simulink model "MPC_stateflow"  (R2018b)
settings: Solver=ode4  StartTime=0.0  StopTime=10  FixedStep=0.01  RelTol=1e-3
values from neighbouring files (symbols this model uses):
  bx0 = 0.4*rand - 0.2    [DataCollection_TrainMPC.m]
  by0 = 0.4*rand - 0.2    [DataCollection_TrainMPC.m]
  bz0 = 0.4*rand - 0.2    [DataCollection_TrainMPC.m]
  px0 = bx0 - (0.1*rand - 0.05)    [DataCollection_TrainMPC.m]
  py0 = by0 - (0.1*rand - 0.05)    [DataCollection_TrainMPC.m]
libraries: neural x148
(part 2 of 5)

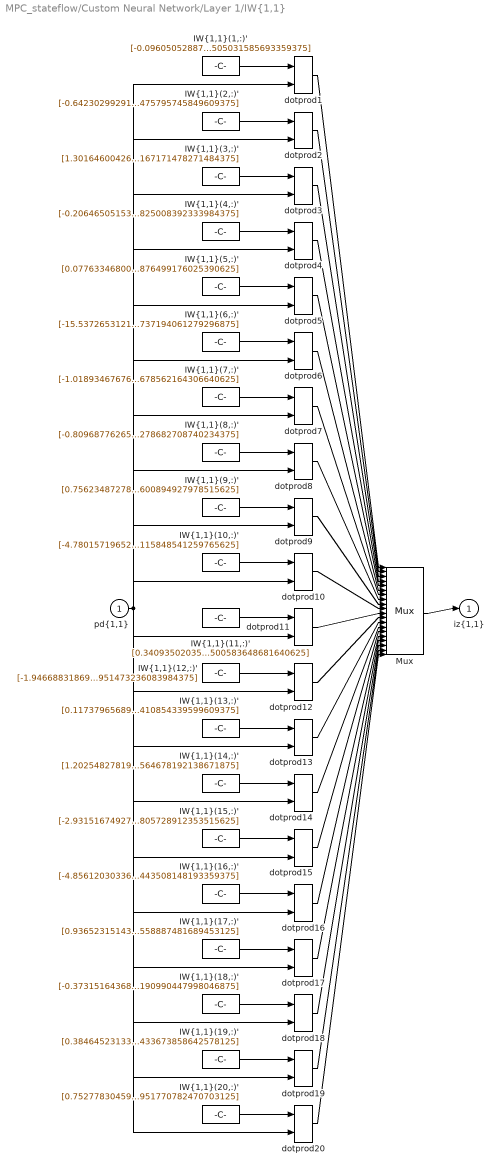
== system MPC_stateflow/Custom Neural Network/Layer 1/IW{1,1} ==
  "pd{1,1}" : Inport  PortDimensions=6
      mask Display: e = 0.06;c1 = [120 230 180]/255;c2 = ([120 230 180]+0)/(256+128);c3 = ([120 230 180]+128)/(256+128);patch([0 1 1 0],[0 0 1 1],c1);patch([0 1 1 1-e 1-e 0+e],[0 0 1 1-e 0+e 0+e],c2);patch([0 0 1 1-e 0+e 0+e],[0 1 1 1-e 1-e 0+e],c3);plot([0 1 1 0 0],[0 0 1 1 0]);
  "IW{1,1}(1,:)'" : Constant  Value=[-0.0960505288717609373438932607314200140535831451416015625;0.831752486119598177793932336498983204364776611328125;-0.0022915027448587575210903199973699884139932692050933837890625;1.253737241349362374620568516547791659832000732421875;1.745603804794473301598145553725771605968475341796875;0.98904804187790629210752513245097361505031585693359375]
      mask Display: e = 0.06;c1 = [120 150 230]/255;c2 = ([120 150 230]+0)/383;c3 = ([120 150 230]+128)/383;patch([0 1 1 0],[0 0 1 1],c1);patch([0 1 1 1-e 1-e 0+e],[0 0 1 1-e 0+e 0+e],c2);patch([0 0 1 1-e 0+e 0+e],[0 1 1 1-e 1-e 0+e],c3);plot([0 1 1 0 0],[0 0 1 1 0]);disp('Weights');
  "IW{1,1}(10,:)'" : Constant  Value=[-4.78015719652584802901174043654464185237884521484375;1.82750965351689753646269309683702886104583740234375;-0.44913035065545636737027734852745197713375091552734375;-0.296705961738857049159179268826846964657306671142578125;1.0273367507350636973484370173537172377109527587890625;-0.76732559429883784307691030335263349115848541259765625]
      mask Display: e = 0.06;c1 = [120 150 230]/255;c2 = ([120 150 230]+0)/383;c3 = ([120 150 230]+128)/383;patch([0 1 1 0],[0 0 1 1],c1);patch([0 1 1 1-e 1-e 0+e],[0 0 1 1-e 0+e 0+e],c2);patch([0 0 1 1-e 0+e 0+e],[0 1 1 1-e 1-e 0+e],c3);plot([0 1 1 0 0],[0 0 1 1 0]);disp('Weights');
  "IW{1,1}(11,:)'" : Constant  Value=[0.3409350203568044523905200549052096903324127197265625;-0.368968737987874106920571648515760898590087890625;-0.8932749097658392312126807155436836183071136474609375;-0.66929160576613444533222718746401369571685791015625;-0.5259460395139445854084669917938299477100372314453125;0.510926105204932756720381803461350500583648681640625]
      mask Display: e = 0.06;c1 = [120 150 230]/255;c2 = ([120 150 230]+0)/383;c3 = ([120 150 230]+128)/383;patch([0 1 1 0],[0 0 1 1],c1);patch([0 1 1 1-e 1-e 0+e],[0 0 1 1-e 0+e 0+e],c2);patch([0 0 1 1-e 0+e 0+e],[0 1 1 1-e 1-e 0+e],c3);plot([0 1 1 0 0],[0 0 1 1 0]);disp('Weights');
  "IW{1,1}(12,:)'" : Constant  Value=[-1.94668831869893121933046131744049489498138427734375;1.8928403055050029291095370354014448821544647216796875;-0.79762269677632680053847025192226283252239227294921875;1.724573381713232489431675276136957108974456787109375;1.37021376275906714425900645437650382518768310546875;-1.2105960555774204490120382615714333951473236083984375]
      mask Display: e = 0.06;c1 = [120 150 230]/255;c2 = ([120 150 230]+0)/383;c3 = ([120 150 230]+128)/383;patch([0 1 1 0],[0 0 1 1],c1);patch([0 1 1 1-e 1-e 0+e],[0 0 1 1-e 0+e 0+e],c2);patch([0 0 1 1-e 0+e 0+e],[0 1 1 1-e 1-e 0+e],c3);plot([0 1 1 0 0],[0 0 1 1 0]);disp('Weights');
  "IW{1,1}(13,:)'" : Constant  Value=[0.1173796568915033144975268442067317664623260498046875;0.6692513437947458232457620397326536476612091064453125;-0.7065428501883797007820930957677774131298065185546875;-0.3044682805089868882220116574899293482303619384765625;0.1473589733445717087079174234531819820404052734375;0.8460490710929666757778022656566463410854339599609375]
      mask Display: e = 0.06;c1 = [120 150 230]/255;c2 = ([120 150 230]+0)/383;c3 = ([120 150 230]+128)/383;patch([0 1 1 0],[0 0 1 1],c1);patch([0 1 1 1-e 1-e 0+e],[0 0 1 1-e 0+e 0+e],c2);patch([0 0 1 1-e 0+e 0+e],[0 1 1 1-e 1-e 0+e],c3);plot([0 1 1 0 0],[0 0 1 1 0]);disp('Weights');
  "IW{1,1}(14,:)'" : Constant  Value=[1.20254827819926735088529312633909285068511962890625;-2.1065505856942312590263099991716444492340087890625;0.66666924060894905412766320296213962137699127197265625;0.0902543188752378544581489450138178654015064239501953125;-1.3922068727151548639398015438928268849849700927734375;0.9483720525673191570348308232496492564678192138671875]
      mask Display: e = 0.06;c1 = [120 150 230]/255;c2 = ([120 150 230]+0)/383;c3 = ([120 150 230]+128)/383;patch([0 1 1 0],[0 0 1 1],c1);patch([0 1 1 1-e 1-e 0+e],[0 0 1 1-e 0+e 0+e],c2);patch([0 0 1 1-e 0+e 0+e],[0 1 1 1-e 1-e 0+e],c3);plot([0 1 1 0 0],[0 0 1 1 0]);disp('Weights');
  "IW{1,1}(15,:)'" : Constant  Value=[-2.931516749274532873670295884949155151844024658203125;0.94843863218748136745261945179663598537445068359375;1.0367786200063264789861250392277725040912628173828125;0.6904689270590800287408228541607968509197235107421875;1.0261103722150346495567418969585560262203216552734375;0.81446211351128694477807812290848232805728912353515625]
      mask Display: e = 0.06;c1 = [120 150 230]/255;c2 = ([120 150 230]+0)/383;c3 = ([120 150 230]+128)/383;patch([0 1 1 0],[0 0 1 1],c1);patch([0 1 1 1-e 1-e 0+e],[0 0 1 1-e 0+e 0+e],c2);patch([0 0 1 1-e 0+e 0+e],[0 1 1 1-e 1-e 0+e],c3);plot([0 1 1 0 0],[0 0 1 1 0]);disp('Weights');
  "IW{1,1}(16,:)'" : Constant  Value=[-4.856120303363926637985059642232954502105712890625;2.2395310961634660174013333744369447231292724609375;-0.74952380593419498655549659815733321011066436767578125;-1.9575546016491471856824091446469537913799285888671875;-0.49184046909802692226776343886740505695343017578125;0.044504062701382872402344759166226140223443508148193359375]
      mask Display: e = 0.06;c1 = [120 150 230]/255;c2 = ([120 150 230]+0)/383;c3 = ([120 150 230]+128)/383;patch([0 1 1 0],[0 0 1 1],c1);patch([0 1 1 1-e 1-e 0+e],[0 0 1 1-e 0+e 0+e],c2);patch([0 0 1 1-e 0+e 0+e],[0 1 1 1-e 1-e 0+e],c3);plot([0 1 1 0 0],[0 0 1 1 0]);disp('Weights');
  "IW{1,1}(17,:)'" : Constant  Value=[0.936523151438795053991270833648741245269775390625;0.4963313087596787909205886535346508026123046875;-0.1718880243608633673346730574849061667919158935546875;0.247344414111217769658424003864638507366180419921875;0.05411620451521859109789147623814642429351806640625;-0.9475780262445614443578278951463289558887481689453125]
      mask Display: e = 0.06;c1 = [120 150 230]/255;c2 = ([120 150 230]+0)/383;c3 = ([120 150 230]+128)/383;patch([0 1 1 0],[0 0 1 1],c1);patch([0 1 1 1-e 1-e 0+e],[0 0 1 1-e 0+e 0+e],c2);patch([0 0 1 1-e 0+e 0+e],[0 1 1 1-e 1-e 0+e],c3);plot([0 1 1 0 0],[0 0 1 1 0]);disp('Weights');
  "IW{1,1}(18,:)'" : Constant  Value=[-0.37315164368151432228160047088749706745147705078125;-0.4391120158711896426240173241239972412586212158203125;0.3888003154554902085493495178525336086750030517578125;0.501884868054674360138278643717058002948760986328125;0.771884198621549000307595633785240352153778076171875;-0.94338702395841078640614796313457190990447998046875]
      mask Display: e = 0.06;c1 = [120 150 230]/255;c2 = ([120 150 230]+0)/383;c3 = ([120 150 230]+128)/383;patch([0 1 1 0],[0 0 1 1],c1);patch([0 1 1 1-e 1-e 0+e],[0 0 1 1-e 0+e 0+e],c2);patch([0 0 1 1-e 0+e 0+e],[0 1 1 1-e 1-e 0+e],c3);plot([0 1 1 0 0],[0 0 1 1 0]);disp('Weights');
  "IW{1,1}(19,:)'" : Constant  Value=[0.38464523133862815740258156438358128070831298828125;0.578558656902977030966894744778983294963836669921875;-0.171641460946194701620015621301718056201934814453125;-0.3022033160443149402141216341988183557987213134765625;-0.2854604799950004601072350851609371602535247802734375;-0.5075778647939082066642413337831385433673858642578125]
      mask Display: e = 0.06;c1 = [120 150 230]/255;c2 = ([120 150 230]+0)/383;c3 = ([120 150 230]+128)/383;patch([0 1 1 0],[0 0 1 1],c1);patch([0 1 1 1-e 1-e 0+e],[0 0 1 1-e 0+e 0+e],c2);patch([0 0 1 1-e 0+e 0+e],[0 1 1 1-e 1-e 0+e],c3);plot([0 1 1 0 0],[0 0 1 1 0]);disp('Weights');
  "IW{1,1}(2,:)'" : Constant  Value=[-0.642302992918277748657374104368500411510467529296875;-0.84943356794090962846865977553534321486949920654296875;0.85502506496665431345860497458488680422306060791015625;0.1584127887998298678251529736371594481170177459716796875;-0.42114165791157687213086546762497164309024810791015625;0.3236613198298134985719798351055942475795745849609375]
      mask Display: e = 0.06;c1 = [120 150 230]/255;c2 = ([120 150 230]+0)/383;c3 = ([120 150 230]+128)/383;patch([0 1 1 0],[0 0 1 1],c1);patch([0 1 1 1-e 1-e 0+e],[0 0 1 1-e 0+e 0+e],c2);patch([0 0 1 1-e 0+e 0+e],[0 1 1 1-e 1-e 0+e],c3);plot([0 1 1 0 0],[0 0 1 1 0]);disp('Weights');
  "IW{1,1}(20,:)'" : Constant  Value=[0.752778304592076619172758000786416232585906982421875;-0.793547986844715946830319808213971555233001708984375;-0.9000930821078256816036855525453574955463409423828125;-0.460144216469947853198618759051896631717681884765625;0.817070301839598389648244847194291651248931884765625;0.7200558973657760208908484855783171951770782470703125]
      mask Display: e = 0.06;c1 = [120 150 230]/255;c2 = ([120 150 230]+0)/383;c3 = ([120 150 230]+128)/383;patch([0 1 1 0],[0 0 1 1],c1);patch([0 1 1 1-e 1-e 0+e],[0 0 1 1-e 0+e 0+e],c2);patch([0 0 1 1-e 0+e 0+e],[0 1 1 1-e 1-e 0+e],c3);plot([0 1 1 0 0],[0 0 1 1 0]);disp('Weights');
  "IW{1,1}(3,:)'" : Constant  Value=[1.301646004268869116771156768663786351680755615234375;-1.57046632470833369410456725745461881160736083984375;-0.049104865692711878455423146760949748568236827850341796875;0.231719255396934553647980692403507418930530548095703125;0.80525102346289945121071696121362037956714630126953125;0.800968281191005271324456771253608167171478271484375]
      mask Display: e = 0.06;c1 = [120 150 230]/255;c2 = ([120 150 230]+0)/383;c3 = ([120 150 230]+128)/383;patch([0 1 1 0],[0 0 1 1],c1);patch([0 1 1 1-e 1-e 0+e],[0 0 1 1-e 0+e 0+e],c2);patch([0 0 1 1-e 0+e 0+e],[0 1 1 1-e 1-e 0+e],c3);plot([0 1 1 0 0],[0 0 1 1 0]);disp('Weights');
  "IW{1,1}(4,:)'" : Constant  Value=[-0.20646505153866012705066168564371764659881591796875;-0.6603391608708621962620100021013058722019195556640625;-0.4244493228273025220431691195699386298656463623046875;0.8891895119816266568335549891344271600246429443359375;0.3268829956368961564550090770353563129901885986328125;0.381793835033847894777636611252091825008392333984375]
      mask Display: e = 0.06;c1 = [120 150 230]/255;c2 = ([120 150 230]+0)/383;c3 = ([120 150 230]+128)/383;patch([0 1 1 0],[0 0 1 1],c1);patch([0 1 1 1-e 1-e 0+e],[0 0 1 1-e 0+e 0+e],c2);patch([0 0 1 1-e 0+e 0+e],[0 1 1 1-e 1-e 0+e],c3);plot([0 1 1 0 0],[0 0 1 1 0]);disp('Weights');
  "IW{1,1}(5,:)'" : Constant  Value=[0.07763346800671389047465709154494106769561767578125;0.7562850068588262697488744379370473325252532958984375;-0.739942855763444651273630370269529521465301513671875;0.1731100810039858384214994657668285071849822998046875;0.243391440418243565346756440703757107257843017578125;0.9946457009029610052408543197088874876499176025390625]
      mask Display: e = 0.06;c1 = [120 150 230]/255;c2 = ([120 150 230]+0)/383;c3 = ([120 150 230]+128)/383;patch([0 1 1 0],[0 0 1 1],c1);patch([0 1 1 1-e 1-e 0+e],[0 0 1 1-e 0+e 0+e],c2);patch([0 0 1 1-e 0+e 0+e],[0 1 1 1-e 1-e 0+e],c3);plot([0 1 1 0 0],[0 0 1 1 0]);disp('Weights');
  "IW{1,1}(6,:)'" : Constant  Value=[-15.5372653121939325870926040806807577610015869140625;3.589611078180853009911288609146140515804290771484375;1.37647289136015427146730871754698455333709716796875;1.5003997535436688348653433422441594302654266357421875;-0.325500014040861429531759085875819437205791473388671875;-3.467041960174273906858388727414421737194061279296875]
      mask Display: e = 0.06;c1 = [120 150 230]/255;c2 = ([120 150 230]+0)/383;c3 = ([120 150 230]+128)/383;patch([0 1 1 0],[0 0 1 1],c1);patch([0 1 1 1-e 1-e 0+e],[0 0 1 1-e 0+e 0+e],c2);patch([0 0 1 1-e 0+e 0+e],[0 1 1 1-e 1-e 0+e],c3);plot([0 1 1 0 0],[0 0 1 1 0]);disp('Weights');
  "IW{1,1}(7,:)'" : Constant  Value=[-1.0189346767621552114491123575135134160518646240234375;0.1768304140142595570761585577201913110911846160888671875;0.322206858111667215904816430338541977107524871826171875;-1.202209597665699458701737967203371226787567138671875;0.73157917366419311644420986340264789760112762451171875;-0.61255466054129359410040933653363026678562164306640625]
      mask Display: e = 0.06;c1 = [120 150 230]/255;c2 = ([120 150 230]+0)/383;c3 = ([120 150 230]+128)/383;patch([0 1 1 0],[0 0 1 1],c1);patch([0 1 1 1-e 1-e 0+e],[0 0 1 1-e 0+e 0+e],c2);patch([0 0 1 1-e 0+e 0+e],[0 1 1 1-e 1-e 0+e],c3);plot([0 1 1 0 0],[0 0 1 1 0]);disp('Weights');
  "IW{1,1}(8,:)'" : Constant  Value=[-0.80968776265257436097755316950497217476367950439453125;0.248817525879779954944837072616792283952236175537109375;0.078067363609808093638520176682504825294017791748046875;-1.8628564188519332045501641914597712457180023193359375;0.06005555953149104009280989657781901769340038299560546875;-0.043826552099953862418058037064838572405278682708740234375]
      mask Display: e = 0.06;c1 = [120 150 230]/255;c2 = ([120 150 230]+0)/383;c3 = ([120 150 230]+128)/383;patch([0 1 1 0],[0 0 1 1],c1);patch([0 1 1 1-e 1-e 0+e],[0 0 1 1-e 0+e 0+e],c2);patch([0 0 1 1-e 0+e 0+e],[0 1 1 1-e 1-e 0+e],c3);plot([0 1 1 0 0],[0 0 1 1 0]);disp('Weights');
  "IW{1,1}(9,:)'" : Constant  Value=[0.756234872781890832271756153204478323459625244140625;0.0663305699460341458006951143033802509307861328125;-0.46890668125554757494910518289543688297271728515625;0.6147825774190476266767291235737502574920654296875;0.1567792287742635348735120714991353452205657958984375;0.3936363229798003349202417666674591600894927978515625]
      mask Display: e = 0.06;c1 = [120 150 230]/255;c2 = ([120 150 230]+0)/383;c3 = ([120 150 230]+128)/383;patch([0 1 1 0],[0 0 1 1],c1);patch([0 1 1 1-e 1-e 0+e],[0 0 1 1-e 0+e 0+e],c2);patch([0 0 1 1-e 0+e 0+e],[0 1 1 1-e 1-e 0+e],c3);plot([0 1 1 0 0],[0 0 1 1 0]);disp('Weights');
  Mux : Mux  Inputs=20
      mask Display: e = 0.06;c1 = [120 150 230]/255;c2 = ([120 150 230]+0)/383;c3 = ([120 150 230]+128)/383;patch([0 1 1 0],[0 0 1 1],c1);patch([0 1 1 1-e 1-e 0+e],[0 0 1 1-e 0+e 0+e],c2);patch([0 0 1 1-e 0+e 0+e],[0 1 1 1-e 1-e 0+e],c3);plot([0 1 1 0 0],[0 0 1 1 0]);disp('Mux');
  dotprod{1..20} (20 alike) : neural/Weight Functions/dotprod
  "iz{1,1}" : Outport
      mask Display: e = 0.06;c1 = [120 230 180]/255;c2 = ([120 230 180]+0)/(256+128);c3 = ([120 230 180]+128)/(256+128);patch([0 1 1 0],[0 0 1 1],c1);patch([0 1 1 1-e 1-e 0+e],[0 0 1 1-e 0+e 0+e],c2);patch([0 0 1 1-e 0+e 0+e],[0 1 1 1-e 1-e 0+e],c3);plot([0 1 1 0 0],[0 0 1 1 0]);
  wires:
  Mux/1 -> "iz{1,1}"/1
  dotprod20/1 -> Mux/20
  "IW{1,1}(20,:)'"/1 -> dotprod20/1
  dotprod19/1 -> Mux/19
  "IW{1,1}(19,:)'"/1 -> dotprod19/1
  dotprod18/1 -> Mux/18
  "IW{1,1}(18,:)'"/1 -> dotprod18/1
  dotprod17/1 -> Mux/17
  "IW{1,1}(17,:)'"/1 -> dotprod17/1
  dotprod16/1 -> Mux/16
  "IW{1,1}(16,:)'"/1 -> dotprod16/1
  dotprod15/1 -> Mux/15
  "IW{1,1}(15,:)'"/1 -> dotprod15/1
  dotprod14/1 -> Mux/14
  "IW{1,1}(14,:)'"/1 -> dotprod14/1
  dotprod13/1 -> Mux/13
  "IW{1,1}(13,:)'"/1 -> dotprod13/1
  dotprod12/1 -> Mux/12
  "IW{1,1}(12,:)'"/1 -> dotprod12/1
  dotprod11/1 -> Mux/11
  "IW{1,1}(11,:)'"/1 -> dotprod11/1
  dotprod10/1 -> Mux/10
  "IW{1,1}(10,:)'"/1 -> dotprod10/1
  dotprod9/1 -> Mux/9
  "IW{1,1}(9,:)'"/1 -> dotprod9/1
  dotprod8/1 -> Mux/8
  "IW{1,1}(8,:)'"/1 -> dotprod8/1
  dotprod7/1 -> Mux/7
  "IW{1,1}(7,:)'"/1 -> dotprod7/1
  dotprod6/1 -> Mux/6
  "IW{1,1}(6,:)'"/1 -> dotprod6/1
  dotprod5/1 -> Mux/5
  "IW{1,1}(5,:)'"/1 -> dotprod5/1
  dotprod4/1 -> Mux/4
  "IW{1,1}(4,:)'"/1 -> dotprod4/1
  dotprod3/1 -> Mux/3
  "IW{1,1}(3,:)'"/1 -> dotprod3/1
  dotprod2/1 -> Mux/2
  "IW{1,1}(2,:)'"/1 -> dotprod2/1
  dotprod1/1 -> Mux/1
  "pd{1,1}"/1 -> dotprod20/2, dotprod19/2, dotprod18/2, dotprod17/2, dotprod16/2, dotprod15/2, dotprod14/2, dotprod13/2, dotprod12/2, dotprod11/2, dotprod10/2, dotprod9/2, dotprod8/2, dotprod7/2, dotprod6/2, dotprod5/2, dotprod4/2, dotprod3/2, dotprod2/2, dotprod1/2
  "IW{1,1}(1,:)'"/1 -> dotprod1/1

== system MPC_stateflow/Custom Neural Network/Layer 2/Delays 1 ==
  "p{2}" : Inport  PortDimensions=20
      mask Display: e = 0.06;c1 = [120 230 180]/255;c2 = ([120 230 180]+0)/(256+128);c3 = ([120 230 180]+128)/(256+128);patch([0 1 1 0],[0 0 1 1],c1);patch([0 1 1 1-e 1-e 0+e],[0 0 1 1-e 0+e 0+e],c2);patch([0 0 1 1-e 0+e 0+e],[0 1 1 1-e 1-e 0+e],c3);plot([0 1 1 0 0],[0 0 1 1 0]);
  mux : Mux  Inputs=1
      mask Display: e = 0.06;c1 = [120 150 230]/255;c2 = ([120 150 230]+0)/383;c3 = ([120 150 230]+128)/383;patch([0 1 1 0],[0 0 1 1],c1);patch([0 1 1 1-e 1-e 0+e],[0 0 1 1-e 0+e 0+e],c2);patch([0 0 1 1-e 0+e 0+e],[0 1 1 1-e 1-e 0+e],c3);plot([0 1 1 0 0],[0 0 1 1 0]);disp('Mux')
  "pd{2,1}" : Outport
      mask Display: e = 0.06;c1 = [120 230 180]/255;c2 = ([120 230 180]+0)/(256+128);c3 = ([120 230 180]+128)/(256+128);patch([0 1 1 0],[0 0 1 1],c1);patch([0 1 1 1-e 1-e 0+e],[0 0 1 1-e 0+e 0+e],c2);patch([0 0 1 1-e 0+e 0+e],[0 1 1 1-e 1-e 0+e],c3);plot([0 1 1 0 0],[0 0 1 1 0]);
  wires:
  mux/1 -> "pd{2,1}"/1
  "p{2}"/1 -> mux/1

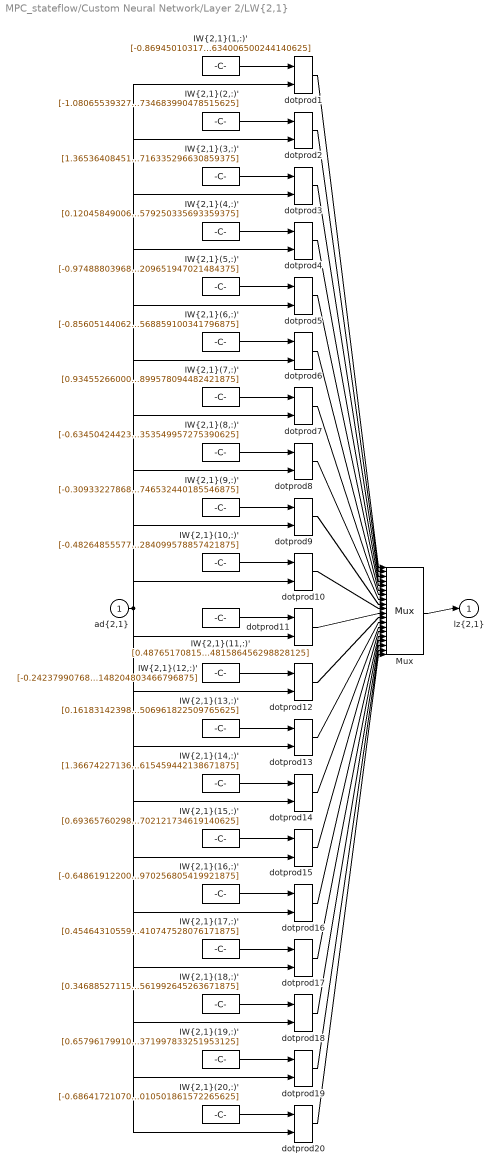
== system MPC_stateflow/Custom Neural Network/Layer 2/LW{2,1} ==
  "ad{2,1}" : Inport  PortDimensions=20
      mask Display: e = 0.06;c1 = [120 230 180]/255;c2 = ([120 230 180]+0)/(256+128);c3 = ([120 230 180]+128)/(256+128);patch([0 1 1 0],[0 0 1 1],c1);patch([0 1 1 1-e 1-e 0+e],[0 0 1 1-e 0+e 0+e],c2);patch([0 0 1 1-e 0+e 0+e],[0 1 1 1-e 1-e 0+e],c3);plot([0 1 1 0 0],[0 0 1 1 0]);
  "IW{2,1}(1,:)'" : Constant  Value=[-0.86945010317003645905487019263091497123241424560546875;-0.9628475956451809647518302881508134305477142333984375;0.464455301408056853151862242157221771776676177978515625;-0.0280186658061805093922203013789840042591094970703125;0.8802149646667343230177493751398287713527679443359375;2.19162758262292101107959751971065998077392578125;-0.2425698325555674383924298354031634517014026641845703125;1.201049187585670363631606960552744567394256591796875;-0.066239954473387374633830404491163790225982666015625;0.369904737379096015814639031304977834224700927734375;0.302608664681982109101454625488258898258209228515625;-0.25611748352890473245935254453797824680805206298828125;-0.4756538324541761397767913877032697200775146484375;1.1118975747010628740696347449556924402713775634765625;-0.66161830384654274350708647034480236470699310302734375;1.1658155789450137529428275229292921721935272216796875;-0.3788254964115800316193372054840438067913055419921875;0.256618075042714277600452987826429307460784912109375;-0.1728271699976773323470524701406247913837432861328125;-0.9351473493710857898264521281816996634006500244140625]
      mask Display: e = 0.06;c1 = [120 150 230]/255;c2 = ([120 150 230]+0)/383;c3 = ([120 150 230]+128)/383;patch([0 1 1 0],[0 0 1 1],c1);patch([0 1 1 1-e 1-e 0+e],[0 0 1 1-e 0+e 0+e],c2);patch([0 0 1 1-e 0+e 0+e],[0 1 1 1-e 1-e 0+e],c3);plot([0 1 1 0 0],[0 0 1 1 0]);disp('weights');
  "IW{2,1}(10,:)'" : Constant  Value=[-0.4826485557719604191362350320559926331043243408203125;-0.531652960170728494659897478413768112659454345703125;1.0598735632520319693838928287732414901256561279296875;-0.7298416839065373640238476582453586161136627197265625;-0.0194929547601445651849871865124441683292388916015625;-0.2250838339207545946152322358102537691593170166015625;0.2295412356918559992902117983248899690806865692138671875;0.2849397026270452659701959419180639088153839111328125;-0.6140745359617743037716763865319080650806427001953125;-0.054128823357529838589119464131726999767124652862548828125;0.2646066348602555962088445085100829601287841796875;-0.94862699481696888259563138490193523466587066650390625;0.1868648989292420736774147371761500835418701171875;0.715345962889761377567765521234832704067230224609375;-0.04799395507758442980250634946060017682611942291259765625;-0.27793384682627542137112186537706293165683746337890625;0.8777729547394266251814087809179909527301788330078125;-0.2574124774418911076878657695488072931766510009765625;0.32820511070958691135501794633455574512481689453125;0.648475679248995628967122684116475284099578857421875]
      mask Display: e = 0.06;c1 = [120 150 230]/255;c2 = ([120 150 230]+0)/383;c3 = ([120 150 230]+128)/383;patch([0 1 1 0],[0 0 1 1],c1);patch([0 1 1 1-e 1-e 0+e],[0 0 1 1-e 0+e 0+e],c2);patch([0 0 1 1-e 0+e 0+e],[0 1 1 1-e 1-e 0+e],c3);plot([0 1 1 0 0],[0 0 1 1 0]);disp('weights');
  "IW{2,1}(11,:)'" : Constant  Value=[0.4876517081501858807968119435827247798442840576171875;0.4906688618130041756870696190162561833858489990234375;0.8639441383936745655347522188094444572925567626953125;0.01132433135379340427562055992893874645233154296875;0.198220615291756718789883962017484009265899658203125;0.6576916159613859225174792300094850361347198486328125;0.3556017828686222070899702885071747004985809326171875;-0.863581303166591762732196002616547048091888427734375;-0.0008316586422278948731445780140347778797149658203125;-0.95533914401638764246627033571712672710418701171875;-0.309405076817836910407777395448647439479827880859375;-0.2669138055125113151433424718561582267284393310546875;0.6876808578623776480043261472019366919994354248046875;-0.315091760312960378342950207297690212726593017578125;-0.19521496028452833826349888113327324390411376953125;0.4636008182845905434277256063069216907024383544921875;-0.9381019874576985717595789537881501019001007080078125;0.8637222332730811746870358547312207520008087158203125;-0.005499813278937448757233141805045306682586669921875;0.2652316335559945503774770259042270481586456298828125]
      mask Display: e = 0.06;c1 = [120 150 230]/255;c2 = ([120 150 230]+0)/383;c3 = ([120 150 230]+128)/383;patch([0 1 1 0],[0 0 1 1],c1);patch([0 1 1 1-e 1-e 0+e],[0 0 1 1-e 0+e 0+e],c2);patch([0 0 1 1-e 0+e 0+e],[0 1 1 1-e 1-e 0+e],c3);plot([0 1 1 0 0],[0 0 1 1 0]);disp('weights');
  "IW{2,1}(12,:)'" : Constant  Value=[-0.2423799076801444185580436396776349283754825592041015625;0.71045454852867617745459938305430114269256591796875;-1.3972510679789784671100960622425191104412078857421875;-0.9569503894516040443107840474112890660762786865234375;-0.968933448898328553156034104176796972751617431640625;6.6339973785591297428254620172083377838134765625;-0.649974583994656018859359392081387341022491455078125;-0.420300460616720938933355000699521042406558990478515625;0.4571713359491924588695610509603284299373626708984375;0.345044005944761755788618984297499991953372955322265625;0.593177356014574996834198827855288982391357421875;1.492063845922114495579080539755523204803466796875;-0.2379677518755716203457950541633181273937225341796875;0.2460320798631776828546691149313119240105152130126953125;2.033348430009402907359117307350970804691314697265625;1.1844441437060206911979776123189367353916168212890625;0.4337573272633783449947486587916500866413116455078125;0.87373676261818733479458387591876089572906494140625;0.038031968147357542164854748989455401897430419921875;0.33746554041346410457435922580771148204803466796875]
      mask Display: e = 0.06;c1 = [120 150 230]/255;c2 = ([120 150 230]+0)/383;c3 = ([120 150 230]+128)/383;patch([0 1 1 0],[0 0 1 1],c1);patch([0 1 1 1-e 1-e 0+e],[0 0 1 1-e 0+e 0+e],c2);patch([0 0 1 1-e 0+e 0+e],[0 1 1 1-e 1-e 0+e],c3);plot([0 1 1 0 0],[0 0 1 1 0]);disp('weights');
  "IW{2,1}(13,:)'" : Constant  Value=[0.1618314239819113875551437331523629836738109588623046875;-0.470160884674381218673033799859695136547088623046875;-0.53793919689711755527383729713619686663150787353515625;0.8959404224353619827780903506209142506122589111328125;0.1869628163932743891706422800780273973941802978515625;0.253487772309714698426574841505498625338077545166015625;-0.1552545568891181282378255446019466035068035125732421875;-0.84467568268962833766266840029857121407985687255859375;-0.583611123182417035337721245014108717441558837890625;0.7376269640629706803025555927888490259647369384765625;-0.107707535993085468106755797634832561016082763671875;0.379956061558021251922667715916759334504604339599609375;0.499716621452286791082997297053225338459014892578125;-0.145456536333087027568211624384275637567043304443359375;-0.92896769722590288864694230142049491405487060546875;-0.202404310214908400578082137144519947469234466552734375;0.7820379085846778099977427700650878250598907470703125;0.688659897131426390615160926245152950286865234375;-0.6505596997821549987151001914753578603267669677734375;-0.046235332957613284321496394113637506961822509765625]
      mask Display: e = 0.06;c1 = [120 150 230]/255;c2 = ([120 150 230]+0)/383;c3 = ([120 150 230]+128)/383;patch([0 1 1 0],[0 0 1 1],c1);patch([0 1 1 1-e 1-e 0+e],[0 0 1 1-e 0+e 0+e],c2);patch([0 0 1 1-e 0+e 0+e],[0 1 1 1-e 1-e 0+e],c3);plot([0 1 1 0 0],[0 0 1 1 0]);disp('weights');
  "IW{2,1}(14,:)'" : Constant  Value=[1.366742271367725525266223485232330858707427978515625;-0.393363022776568704852451219267095439136028289794921875;0.35963396200540775904386237016296945512294769287109375;0.654230942341464949407736639841459691524505615234375;-0.1326473020210834352639039934729225933551788330078125;-3.28762404715274403343983067316003143787384033203125;-0.0911863455292211411151725997115136124193668365478515625;-0.350368599710001671354575591976754367351531982421875;-0.5039328832455385320798768589156679809093475341796875;0.509101395846049076254757892456836998462677001953125;0.5654988295683438526140207613934762775897979736328125;1.1192035066205392457305833886493928730487823486328125;0.022282956594256386750885212677530944347381591796875;0.10840420140515542868353549010862479917705059051513671875;0.96883348602309471431226484128274023532867431640625;-0.50278354234049416060514658965985290706157684326171875;-0.9454255529650623657289543189108371734619140625;0.8404130286113209447051985989673994481563568115234375;0.1414317030925127394169749095453880727291107177734375;-0.97372728615385550909877565572969615459442138671875]
      mask Display: e = 0.06;c1 = [120 150 230]/255;c2 = ([120 150 230]+0)/383;c3 = ([120 150 230]+128)/383;patch([0 1 1 0],[0 0 1 1],c1);patch([0 1 1 1-e 1-e 0+e],[0 0 1 1-e 0+e 0+e],c2);patch([0 0 1 1-e 0+e 0+e],[0 1 1 1-e 1-e 0+e],c3);plot([0 1 1 0 0],[0 0 1 1 0]);disp('weights');
  "IW{2,1}(15,:)'" : Constant  Value=[0.6936576029800705089911616596509702503681182861328125;-0.25983160417178741141697173588909208774566650390625;0.8980326413752328651440848261700011789798736572265625;-0.969962038515755242684690529131330549716949462890625;0.6147210577696828881499868657556362450122833251953125;0.1736666813121658936580615772982127964496612548828125;0.5952776079171331335970762665965594351291656494140625;-0.636774297338472461404990099254064261913299560546875;0.70334374987273395873899062280543148517608642578125;0.07688118518908737542005837894976139068603515625;0.9809435672476813916631499523646198213100433349609375;-0.6227263980893782413517101304023526608943939208984375;0.08190360992437728526738283107988536357879638671875;0.2529923172485875060289117755019105970859527587890625;-0.748717237724522366448809407302178442478179931640625;-0.653139658425754277004671166650950908660888671875;0.04410249450502146117969459737651050090789794921875;-0.544199420097366104442926371120847761631011962890625;0.993506850416419950988711207173764705657958984375;-0.2939878289163504465619780603446997702121734619140625]
      mask Display: e = 0.06;c1 = [120 150 230]/255;c2 = ([120 150 230]+0)/383;c3 = ([120 150 230]+128)/383;patch([0 1 1 0],[0 0 1 1],c1);patch([0 1 1 1-e 1-e 0+e],[0 0 1 1-e 0+e 0+e],c2);patch([0 0 1 1-e 0+e 0+e],[0 1 1 1-e 1-e 0+e],c3);plot([0 1 1 0 0],[0 0 1 1 0]);disp('weights');
  "IW{2,1}(16,:)'" : Constant  Value=[-0.64861912200991234112024130809004418551921844482421875;0.721480501821621711400212006992660462856292724609375;0.32699986582939588597440661033033393323421478271484375;-0.6476074888498895010258138427161611616611480712890625;-0.369510393809254100716543689486570656299591064453125;1.246805620640468514892518214765004813671112060546875;1.219610087621920246903073348221369087696075439453125;0.1662383984196948716327568718043039552867412567138671875;-0.1683025634649453206037605923484079539775848388671875;1.535647982148657941792180281481705605983734130859375;-0.3995033209321998679541820820304565131664276123046875;0.06036852059349755161843376072283717803657054901123046875;0.918868642123504830721003600046969950199127197265625;-1.2901867078027933199990684443037025630474090576171875;0.780400069817255737092409617616795003414154052734375;0.1990641497121203029596614442198188044130802154541015625;-0.34802037645994943204641458578407764434814453125;-0.8250355808928182543837692719534970819950103759765625;0.633670217583243822190297578345052897930145263671875;-0.0158563970128831055461660071159712970256805419921875]
      mask Display: e = 0.06;c1 = [120 150 230]/255;c2 = ([120 150 230]+0)/383;c3 = ([120 150 230]+128)/383;patch([0 1 1 0],[0 0 1 1],c1);patch([0 1 1 1-e 1-e 0+e],[0 0 1 1-e 0+e 0+e],c2);patch([0 0 1 1-e 0+e 0+e],[0 1 1 1-e 1-e 0+e],c3);plot([0 1 1 0 0],[0 0 1 1 0]);disp('weights');
  "IW{2,1}(17,:)'" : Constant  Value=[0.45464310559893561514144266766379587352275848388671875;0.4529374704014650365735406012390740215778350830078125;-0.75921684877630790655445025549852289259433746337890625;-0.33587285126632604459473441238515079021453857421875;0.785777417050302684486950965947471559047698974609375;9.3449961980014517592962874914519488811492919921875;1.6409870586549715198998455889523029327392578125;0.578457000499050355557528746430762112140655517578125;0.233370134310472376881762102129869163036346435546875;2.92359285650911271403629143605940043926239013671875;-0.7139883434838012465917245208402164280414581298828125;-0.10755020807965987028609333719941787421703338623046875;0.6079217829972936026905472317594103515148162841796875;-1.1541763575095778104895316573674790561199188232421875;1.0201769917919698560382357754861004650592803955078125;2.280579523437183286915796998073346912860870361328125;0.718978641731171652651255499222315847873687744140625;-0.54538052743062248595151686458848416805267333984375;0.1887452476619555508108305730274878442287445068359375;0.4601824221802086611887716571800410747528076171875]
      mask Display: e = 0.06;c1 = [120 150 230]/255;c2 = ([120 150 230]+0)/383;c3 = ([120 150 230]+128)/383;patch([0 1 1 0],[0 0 1 1],c1);patch([0 1 1 1-e 1-e 0+e],[0 0 1 1-e 0+e 0+e],c2);patch([0 0 1 1-e 0+e 0+e],[0 1 1 1-e 1-e 0+e],c3);plot([0 1 1 0 0],[0 0 1 1 0]);disp('weights');
  "IW{2,1}(18,:)'" : Constant  Value=[0.346885271156239516354702345779514871537685394287109375;0.348093907222798815137565497934701852500438690185546875;0.7381264553490314295203233996289782226085662841796875;-0.7380063103781662192659496213309466838836669921875;0.1557144305690709717993058802676387131214141845703125;2.367869383175240205474665344809181988239288330078125;-0.118973993123826726758807126316241919994354248046875;0.457037682108792753243875495172687806189060211181640625;-0.532667721521499881731642744853161275386810302734375;0.46675155999001127771208530248259194195270538330078125;0.80261687269854764537058144924230873584747314453125;1.451894766366281341873900601058267056941986083984375;-0.9353538667528520367255850942456163465976715087890625;-1.1424264474399457025555193467880599200725555419921875;0.1606066022159286232895425428068847395479679107666015625;-1.0421273903774366242913629321265034377574920654296875;0.11703310184503568081026969593949615955352783203125;-0.371246767771899133236956913606263697147369384765625;0.951978136661809859475624762126244604587554931640625;-0.0627433145077815890289230082998983561992645263671875]
      mask Display: e = 0.06;c1 = [120 150 230]/255;c2 = ([120 150 230]+0)/383;c3 = ([120 150 230]+128)/383;patch([0 1 1 0],[0 0 1 1],c1);patch([0 1 1 1-e 1-e 0+e],[0 0 1 1-e 0+e 0+e],c2);patch([0 0 1 1-e 0+e 0+e],[0 1 1 1-e 1-e 0+e],c3);plot([0 1 1 0 0],[0 0 1 1 0]);disp('weights');
  "IW{2,1}(19,:)'" : Constant  Value=[0.6579617991003574584141233572154305875301361083984375;-0.866927037291770119509237702004611492156982421875;0.2831324178926750700924230841337703168392181396484375;0.618981384253164179654049803502857685089111328125;-0.6319795967450698714884538276237435638904571533203125;0.3961144968946059830017247804789803922176361083984375;-0.4595834759404844316321714359219186007976531982421875;0.1389888254907514220093389667454175651073455810546875;-0.7960654811484051407433071290142834186553955078125;0.7082308876730774027663528613629750907421112060546875;0.0831187577747465322630660011782310903072357177734375;-0.5921875495337562966824407340027391910552978515625;0.418774502462590181295354341273196041584014892578125;-0.866550004721287070452717671287246048450469970703125;-0.9939640867608072749561642922344617545604705810546875;-0.47140503454619864243113624979741871356964111328125;0.380455736325495674776675514294765889644622802734375;-0.650468247287376843956963057280518114566802978515625;0.8031251693386425305476450375863350927829742431640625;-0.0851901678211366419901651170221157371997833251953125]
      mask Display: e = 0.06;c1 = [120 150 230]/255;c2 = ([120 150 230]+0)/383;c3 = ([120 150 230]+128)/383;patch([0 1 1 0],[0 0 1 1],c1);patch([0 1 1 1-e 1-e 0+e],[0 0 1 1-e 0+e 0+e],c2);patch([0 0 1 1-e 0+e 0+e],[0 1 1 1-e 1-e 0+e],c3);plot([0 1 1 0 0],[0 0 1 1 0]);disp('weights');
  "IW{2,1}(2,:)'" : Constant  Value=[-1.0806553932786810978683433859259821474552154541015625;-0.859955712561555341011398923001252114772796630859375;-0.81143099224970594018913061518105678260326385498046875;0.2086209658399464927924782386980950832366943359375;0.1640283598941600917697769546066410839557647705078125;-1.23271399361495515023534608189947903156280517578125;0.56672855173635083847472060369909740984439849853515625;0.48456887902243217514097750608925707638263702392578125;-0.309655897689570025477223680354654788970947265625;-0.6057893011983217501637000168557278811931610107421875;0.4070339763053059112252185514080338180065155029296875;0.12454988425188946721267058137527783401310443878173828125;0.50034482659598555898128324770368635654449462890625;-0.1687741106642130783921373904377105645835399627685546875;-1.359239838595867500004032990545965731143951416015625;0.82329734513879271329273024093708954751491546630859375;0.9648348985858856696751217896235175430774688720703125;-0.419806296625148345214029177441261708736419677734375;0.6327030236544282093547053591464646160602569580078125;-0.8128458083650385024299112046719528734683990478515625]
      mask Display: e = 0.06;c1 = [120 150 230]/255;c2 = ([120 150 230]+0)/383;c3 = ([120 150 230]+128)/383;patch([0 1 1 0],[0 0 1 1],c1);patch([0 1 1 1-e 1-e 0+e],[0 0 1 1-e 0+e 0+e],c2);patch([0 0 1 1-e 0+e 0+e],[0 1 1 1-e 1-e 0+e],c3);plot([0 1 1 0 0],[0 0 1 1 0]);disp('weights');
  "IW{2,1}(20,:)'" : Constant  Value=[-0.6864172107078314599704071952146477997303009033203125;-0.479369802842918080187928353552706539630889892578125;-0.2199845717175075154870000915252603590488433837890625;-0.3105266946334130917506399782723747193813323974609375;0.5758584676510085653688975071418099105358123779296875;0.7289588601091996356018398728338070213794708251953125;-0.4952665969908205401139866808080114424228668212890625;-0.678057126368782459024941999814473092555999755859375;0.0317140339370596269219504392822273075580596923828125;-0.802513196359303293547782232053577899932861328125;0.9494807417101644997359244371182285249233245849609375;-0.504534196475290297456695043365471065044403076171875;-0.0699970368729878611446793001960031688213348388671875;-0.0828323725831363599780843287589959800243377685546875;0.9023875709804090039511947907158173620700836181640625;0.638178357267061624469306480023078620433807373046875;-0.094293000096925094766220354358665645122528076171875;0.2141883239449209330729217981570400297641754150390625;0.1912158672052910457495045193354599177837371826171875;-0.7246745181087936860109266490326263010501861572265625]
      mask Display: e = 0.06;c1 = [120 150 230]/255;c2 = ([120 150 230]+0)/383;c3 = ([120 150 230]+128)/383;patch([0 1 1 0],[0 0 1 1],c1);patch([0 1 1 1-e 1-e 0+e],[0 0 1 1-e 0+e 0+e],c2);patch([0 0 1 1-e 0+e 0+e],[0 1 1 1-e 1-e 0+e],c3);plot([0 1 1 0 0],[0 0 1 1 0]);disp('weights');
  "IW{2,1}(3,:)'" : Constant  Value=[1.3653640845112018364915229540201835334300994873046875;0.306765011951229793485396157848299480974674224853515625;0.020793587999859898529653179366505355574190616607666015625;0.099095843017125151419577377964742481708526611328125;0.7576639688236881386984578057308681309223175048828125;3.3203980492572231497661050525493919849395751953125;0.051763083102982075656139926422838470898568630218505859375;0.341073559737574416583782976886141113936901092529296875;-0.5499200843718308195917643388384021818637847900390625;1.5318590406784975410658944383612833917140960693359375;0.22048162529325932013080091564916074275970458984375;0.820735541014840919160633347928524017333984375;-0.0860493451286143962164487675181590020656585693359375;-1.0167176992358555320805635346914641559123992919921875;1.6964552720312353617515555015415884554386138916015625;1.79534049531465367266491739428602159023284912109375;-0.466722595696729580794226421858184039592742919921875;-0.9813028440669684382413606726913712918758392333984375;-0.62973920346193867914053043932653963565826416015625;-0.869256569915547228077912222943268716335296630859375]
      mask Display: e = 0.06;c1 = [120 150 230]/255;c2 = ([120 150 230]+0)/383;c3 = ([120 150 230]+128)/383;patch([0 1 1 0],[0 0 1 1],c1);patch([0 1 1 1-e 1-e 0+e],[0 0 1 1-e 0+e 0+e],c2);patch([0 0 1 1-e 0+e 0+e],[0 1 1 1-e 1-e 0+e],c3);plot([0 1 1 0 0],[0 0 1 1 0]);disp('weights');
  "IW{2,1}(4,:)'" : Constant  Value=[0.1204584900671190894616557898189057596027851104736328125;-0.2802269618452044586121019165148027241230010986328125;0.2472333569965907695831219825777225196361541748046875;0.852362853412907295336253810091875493526458740234375;0.689468890784443733110720131662674248218536376953125;0.007761819150829019943460540531532387831248342990875244140625;-0.7987799736009602025177400719258002936840057373046875;0.5636780929170390752602770589874126017093658447265625;0.1850237375315935128838873424683697521686553955078125;-0.432454595119342533049433541236794553697109222412109375;0.5992305234720560758177043680916540324687957763671875;0.0219114806932921568627392616690485738217830657958984375;-0.886141123177810019484468284645117819309234619140625;-0.72251917139723842442577961264760233461856842041015625;-0.71985290991653083647605626538279466331005096435546875;-1.275377001876238924893414150574244558811187744140625;0.0673066899424228370918399377842433750629425048828125;0.153511869974181536235846579074859619140625;0.4037530595126208599054962178342975676059722900390625;-0.096533702617049410577010348788462579250335693359375]
      mask Display: e = 0.06;c1 = [120 150 230]/255;c2 = ([120 150 230]+0)/383;c3 = ([120 150 230]+128)/383;patch([0 1 1 0],[0 0 1 1],c1);patch([0 1 1 1-e 1-e 0+e],[0 0 1 1-e 0+e 0+e],c2);patch([0 0 1 1-e 0+e 0+e],[0 1 1 1-e 1-e 0+e],c3);plot([0 1 1 0 0],[0 0 1 1 0]);disp('weights');
  "IW{2,1}(5,:)'" : Constant  Value=[-0.9748880396817682925103554225643165409564971923828125;0.1377028741729626748480086462222971022129058837890625;0.8496159407987013967300526928738690912723541259765625;0.8374668712672121984041950781829655170440673828125;0.81078463741729844826977569027803838253021240234375;0.8372035559550516925497731790528632700443267822265625;-0.1783773001556288040347908463445492088794708251953125;0.4662850505750222307455032932921312749385833740234375;-0.3754603245961660729079767406801693141460418701171875;0.308274693941488653337046343949623405933380126953125;-0.9308575602567314977164869560510851442813873291015625;-0.729144193855660205372259952127933502197265625;0.0170324812204791786740543102496303617954254150390625;-0.1427623426724269339871398187824524939060211181640625;0.493876991215050242800543855992145836353302001953125;-0.684539860258933430259276065044105052947998046875;-0.37106597762830073605755387688986957073211669921875;-0.3771115717350743690161607446498237550258636474609375;-0.5192887503017222794454710310674272477626800537109375;-0.2491303336642844978854327564476989209651947021484375]
      mask Display: e = 0.06;c1 = [120 150 230]/255;c2 = ([120 150 230]+0)/383;c3 = ([120 150 230]+128)/383;patch([0 1 1 0],[0 0 1 1],c1);patch([0 1 1 1-e 1-e 0+e],[0 0 1 1-e 0+e 0+e],c2);patch([0 0 1 1-e 0+e 0+e],[0 1 1 1-e 1-e 0+e],c3);plot([0 1 1 0 0],[0 0 1 1 0]);disp('weights');
  "IW{2,1}(6,:)'" : Constant  Value=[-0.8560514406210264493068962110555730760097503662109375;-0.36527518135567849100198145606555044651031494140625;-0.473406459025778048044230672530829906463623046875;-0.21024877415289022764000037568621337413787841796875;-0.0802394683663860686095858909538947045803070068359375;-0.999195950217285133732048052479512989521026611328125;-0.197040833060918796348914838745258748531341552734375;0.0380232549281116494199750377447344362735748291015625;0.8326111069367014838604745818884111940860748291015625;-0.710908919750680379223695126711390912532806396484375;0.54047746910995986269199420348741114139556884765625;-0.2885896580322377946714595964294858276844024658203125;-0.576079670712648095332042430527508258819580078125;-0.7819624719618634145490432274527847766876220703125;-0.095190346507096901262912069796584546566009521484375;-0.6247366541951320240144696072093211114406585693359375;0.82154566234767489874002421856857836246490478515625;0.0345351970022595988751845652586780488491058349609375;0.1484381776817194076301120730931870639324188232421875;0.950700068540573095532408842700533568859100341796875]
      mask Display: e = 0.06;c1 = [120 150 230]/255;c2 = ([120 150 230]+0)/383;c3 = ([120 150 230]+128)/383;patch([0 1 1 0],[0 0 1 1],c1);patch([0 1 1 1-e 1-e 0+e],[0 0 1 1-e 0+e 0+e],c2);patch([0 0 1 1-e 0+e 0+e],[0 1 1 1-e 1-e 0+e],c3);plot([0 1 1 0 0],[0 0 1 1 0]);disp('weights');
  "IW{2,1}(7,:)'" : Constant  Value=[0.93455266000054404429420173983089625835418701171875;0.9772323088248977551728557955357246100902557373046875;-0.868077818631952435879384211148135364055633544921875;0.9265250568814236142856088918051682412624359130859375;0.09269363204074654305486546945758163928985595703125;0.953518298062119296076843966147862374782562255859375;-0.3652321080834461941577728794072754681110382080078125;0.5417678210037759622963449146482162177562713623046875;0.81927104990311416798931531957350671291351318359375;0.5030556342704877170746158299152739346027374267578125;0.4634572014790538929673857637681066989898681640625;-0.947562865407253429594902627286501228809356689453125;0.597208489520420382490328847779892385005950927734375;0.267573521223835708582328152260743081569671630859375;-0.0998265059984777547441581191378645598888397216796875;0.2449918045998422666542637671227566897869110107421875;-0.266886712297531136783845795434899628162384033203125;0.8328117061077955352033086455776356160640716552734375;-0.3020248055584222601765986837563104927539825439453125;-0.6640334136007701726356344806845299899578094482421875]
      mask Display: e = 0.06;c1 = [120 150 230]/255;c2 = ([120 150 230]+0)/383;c3 = ([120 150 230]+128)/383;patch([0 1 1 0],[0 0 1 1],c1);patch([0 1 1 1-e 1-e 0+e],[0 0 1 1-e 0+e 0+e],c2);patch([0 0 1 1-e 0+e 0+e],[0 1 1 1-e 1-e 0+e],c3);plot([0 1 1 0 0],[0 0 1 1 0]);disp('weights');
  "IW{2,1}(8,:)'" : Constant  Value=[-0.6345042442310167007946120065753348171710968017578125;-0.4717527842355411227259764928021468222141265869140625;0.788463567668844955704798849183134734630584716796875;-0.6520886666390712793628381405142135918140411376953125;0.5972071823040787652558947229408659040927886962890625;-3.374925678704658427164986278512515127658843994140625;0.13502919411089220336208427397650666534900665283203125;1.25348702649655052709931624121963977813720703125;-0.4857634124356076110728963612928055226802825927734375;-1.2010723698476957199687831234768964350223541259765625;-0.4806032134032938163414883092627860605716705322265625;-2.00595393766520135869768637348897755146026611328125;-0.40533723698545554015026937122456729412078857421875;1.560418682388652111825422252877615392208099365234375;-1.460816286938797947669854693231172859668731689453125;0.3312299944520813443915585594368167221546173095703125;-0.13281534545367090771605944610200822353363037109375;-0.14705042299720805232254861039109528064727783203125;-0.8860712010343345657048530483734793961048126220703125;0.9455751838653103646947784000076353549957275390625]
      mask Display: e = 0.06;c1 = [120 150 230]/255;c2 = ([120 150 230]+0)/383;c3 = ([120 150 230]+128)/383;patch([0 1 1 0],[0 0 1 1],c1);patch([0 1 1 1-e 1-e 0+e],[0 0 1 1-e 0+e 0+e],c2);patch([0 0 1 1-e 0+e 0+e],[0 1 1 1-e 1-e 0+e],c3);plot([0 1 1 0 0],[0 0 1 1 0]);disp('weights');
  "IW{2,1}(9,:)'" : Constant  Value=[-0.309332278688601636229549285417306236922740936279296875;0.26532456401708504056813353599864058196544647216796875;0.07769485023417209423879370433496660552918910980224609375;-0.7473409611207253444575826506479643285274505615234375;-0.428562296531704856050737362238578498363494873046875;6.5625484154600304265159138594754040241241455078125;0.347191720226565525564410563674755394458770751953125;0.09995430888087193654900630690463003702461719512939453125;-0.7782173985119416048661378226825036108493804931640625;1.272310780555977682837465181364677846431732177734375;-0.4858614023557066285974315178464166820049285888671875;0.2240247267275335685265957863521180115640163421630859375;-0.9447879760909927426837384700775146484375;0.31331997050244708713506724961916916072368621826171875;1.04865363300881053731927750050090253353118896484375;1.85888278982414067996842277352698147296905517578125;0.0245853845567227669022258851327933371067047119140625;-0.5052079267952291896648375768563710153102874755859375;-0.542372658079248282092521549202501773834228515625;0.53494973772602616435278832796029746532440185546875]
      mask Display: e = 0.06;c1 = [120 150 230]/255;c2 = ([120 150 230]+0)/383;c3 = ([120 150 230]+128)/383;patch([0 1 1 0],[0 0 1 1],c1);patch([0 1 1 1-e 1-e 0+e],[0 0 1 1-e 0+e 0+e],c2);patch([0 0 1 1-e 0+e 0+e],[0 1 1 1-e 1-e 0+e],c3);plot([0 1 1 0 0],[0 0 1 1 0]);disp('weights');
  Mux : Mux  Inputs=20
      mask Display: e = 0.06;c1 = [120 150 230]/255;c2 = ([120 150 230]+0)/383;c3 = ([120 150 230]+128)/383;patch([0 1 1 0],[0 0 1 1],c1);patch([0 1 1 1-e 1-e 0+e],[0 0 1 1-e 0+e 0+e],c2);patch([0 0 1 1-e 0+e 0+e],[0 1 1 1-e 1-e 0+e],c3);plot([0 1 1 0 0],[0 0 1 1 0]);disp('Mux');
  dotprod{1..20} (20 alike) : neural/Weight Functions/dotprod
  "lz{2,1}" : Outport
      mask Display: e = 0.06;c1 = [120 230 180]/255;c2 = ([120 230 180]+0)/(256+128);c3 = ([120 230 180]+128)/(256+128);patch([0 1 1 0],[0 0 1 1],c1);patch([0 1 1 1-e 1-e 0+e],[0 0 1 1-e 0+e 0+e],c2);patch([0 0 1 1-e 0+e 0+e],[0 1 1 1-e 1-e 0+e],c3);plot([0 1 1 0 0],[0 0 1 1 0]);
  wires:
  Mux/1 -> "lz{2,1}"/1
  dotprod20/1 -> Mux/20
  "IW{2,1}(20,:)'"/1 -> dotprod20/1
  dotprod19/1 -> Mux/19
  "IW{2,1}(19,:)'"/1 -> dotprod19/1
  dotprod18/1 -> Mux/18
  "IW{2,1}(18,:)'"/1 -> dotprod18/1
  dotprod17/1 -> Mux/17
  "IW{2,1}(17,:)'"/1 -> dotprod17/1
  dotprod16/1 -> Mux/16
  "IW{2,1}(16,:)'"/1 -> dotprod16/1
  dotprod15/1 -> Mux/15
  "IW{2,1}(15,:)'"/1 -> dotprod15/1
  dotprod14/1 -> Mux/14
  "IW{2,1}(14,:)'"/1 -> dotprod14/1
  dotprod13/1 -> Mux/13
  "IW{2,1}(13,:)'"/1 -> dotprod13/1
  dotprod12/1 -> Mux/12
  "IW{2,1}(12,:)'"/1 -> dotprod12/1
  dotprod11/1 -> Mux/11
  "IW{2,1}(11,:)'"/1 -> dotprod11/1
  dotprod10/1 -> Mux/10
  "IW{2,1}(10,:)'"/1 -> dotprod10/1
  dotprod9/1 -> Mux/9
  "IW{2,1}(9,:)'"/1 -> dotprod9/1
  dotprod8/1 -> Mux/8
  "IW{2,1}(8,:)'"/1 -> dotprod8/1
  dotprod7/1 -> Mux/7
  "IW{2,1}(7,:)'"/1 -> dotprod7/1
  dotprod6/1 -> Mux/6
  "IW{2,1}(6,:)'"/1 -> dotprod6/1
  dotprod5/1 -> Mux/5
  "IW{2,1}(5,:)'"/1 -> dotprod5/1
  dotprod4/1 -> Mux/4
  "IW{2,1}(4,:)'"/1 -> dotprod4/1
  dotprod3/1 -> Mux/3
  "IW{2,1}(3,:)'"/1 -> dotprod3/1
  dotprod2/1 -> Mux/2
  "IW{2,1}(2,:)'"/1 -> dotprod2/1
  dotprod1/1 -> Mux/1
  "ad{2,1}"/1 -> dotprod20/2, dotprod19/2, dotprod18/2, dotprod17/2, dotprod16/2, dotprod15/2, dotprod14/2, dotprod13/2, dotprod12/2, dotprod11/2, dotprod10/2, dotprod9/2, dotprod8/2, dotprod7/2, dotprod6/2, dotprod5/2, dotprod4/2, dotprod3/2, dotprod2/2, dotprod1/2
  "IW{2,1}(1,:)'"/1 -> dotprod1/1

== system MPC_stateflow/Custom Neural Network/Layer 3/Delays 1 ==
  "p{3}" : Inport  PortDimensions=20
      mask Display: e = 0.06;c1 = [120 230 180]/255;c2 = ([120 230 180]+0)/(256+128);c3 = ([120 230 180]+128)/(256+128);patch([0 1 1 0],[0 0 1 1],c1);patch([0 1 1 1-e 1-e 0+e],[0 0 1 1-e 0+e 0+e],c2);patch([0 0 1 1-e 0+e 0+e],[0 1 1 1-e 1-e 0+e],c3);plot([0 1 1 0 0],[0 0 1 1 0]);
  mux : Mux  Inputs=1
      mask Display: e = 0.06;c1 = [120 150 230]/255;c2 = ([120 150 230]+0)/383;c3 = ([120 150 230]+128)/383;patch([0 1 1 0],[0 0 1 1],c1);patch([0 1 1 1-e 1-e 0+e],[0 0 1 1-e 0+e 0+e],c2);patch([0 0 1 1-e 0+e 0+e],[0 1 1 1-e 1-e 0+e],c3);plot([0 1 1 0 0],[0 0 1 1 0]);disp('Mux')
  "pd{3,2}" : Outport
      mask Display: e = 0.06;c1 = [120 230 180]/255;c2 = ([120 230 180]+0)/(256+128);c3 = ([120 230 180]+128)/(256+128);patch([0 1 1 0],[0 0 1 1],c1);patch([0 1 1 1-e 1-e 0+e],[0 0 1 1-e 0+e 0+e],c2);patch([0 0 1 1-e 0+e 0+e],[0 1 1 1-e 1-e 0+e],c3);plot([0 1 1 0 0],[0 0 1 1 0]);
  wires:
  mux/1 -> "pd{3,2}"/1
  "p{3}"/1 -> mux/1
